simulink model "m7_2_simulink"  (R2019a)
settings: Solver=VariableStepAuto  StartTime=0.0  StopTime=10.0  RelTol=1e-3
settings Model: Creator=liang  LastModifiedBy=liang

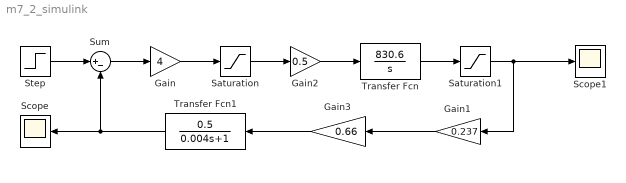
== system m7_2_simulink ==
  Gain : Gain  Gain=4
  Gain1 : Gain  Gain=0.237
  Gain2 : Gain  Gain=0.5
  Gain3 : Gain  Gain=0.66
  Saturation : Saturate  UpperLimit=11  LowerLimit=-11
  Saturation1 : Saturate  UpperLimit=120  LowerLimit=-120
  Scope : Scope
  Scope1 : Scope
  Step : Step  SampleTime=0
  Sum : Sum  Inputs=|+-
  Transfer Fcn : TransferFcn  Numerator=[830.6]  Denominator=[1 0]
  Transfer Fcn1 : TransferFcn  Numerator=[0.5]  Denominator=[0.004 1]
  wires:
  Sum/1 -> Gain/1
  Gain1/1 -> Gain3/1
  Transfer Fcn1/1 -> Scope/1, Sum/2
  Gain3/1 -> Transfer Fcn1/1
  Saturation/1 -> Gain2/1
  Gain2/1 -> Transfer Fcn/1
  Transfer Fcn/1 -> Saturation1/1
  Step/1 -> Sum/1
  Gain/1 -> Saturation/1
  Saturation1/1 -> Scope1/1, Gain1/1
